simulink model "BoostQSim2018a"  (R2018a)
settings: Solver=VariableStepAuto  StartTime=0.0  StopTime=Tsim  RelTol=1e-3
values from neighbouring files (symbols this model uses):
  BoostQ =     [Boost_Data.mat]
  BoostQParam =     [BoostQParameters.mat]
  DutyConst = BoostQParam.Dn    [BoostQ.m]
  Gains =     [Gains.mat]
  PRBS_Amp = .05    (= 0.05)    [BoostQ.m]    (also in BoostQPlms.m = 0.1; BoostQuadrat.m; QBoostPLMS.m)
  PRBS_N = 10    [BoostQ.m]    (also in BoostQPlms.m; BoostQuadrat.m; QBoostPLMS.m)
  PRBS_Ts = Tb    (= 0.002)    [BoostQ.m]    (also in BoostQPlms.m; BoostQuadrat.m; QBoostPLMS.m)
  Ramp_Max = 0.75    [BoostQ.m]    (also in BoostQPlms.m; BoostQuadrat.m; QBoostPLMS.m)
  Tsim = 1*Tsim_min    (= 2.046)    [BoostQ.m]    (also in BoostQPlms.m; BoostQuadrat.m; QBoostPLMS.m)
undefined symbols (not defined in the file or in its folder): RST_LPV, Unit
libraries: fl_lib x11, nesl_utility x8, pe_lib x5, powerlib_meascontrol x1
settings Model: Creator=marcus  LastModifiedBy=projeto

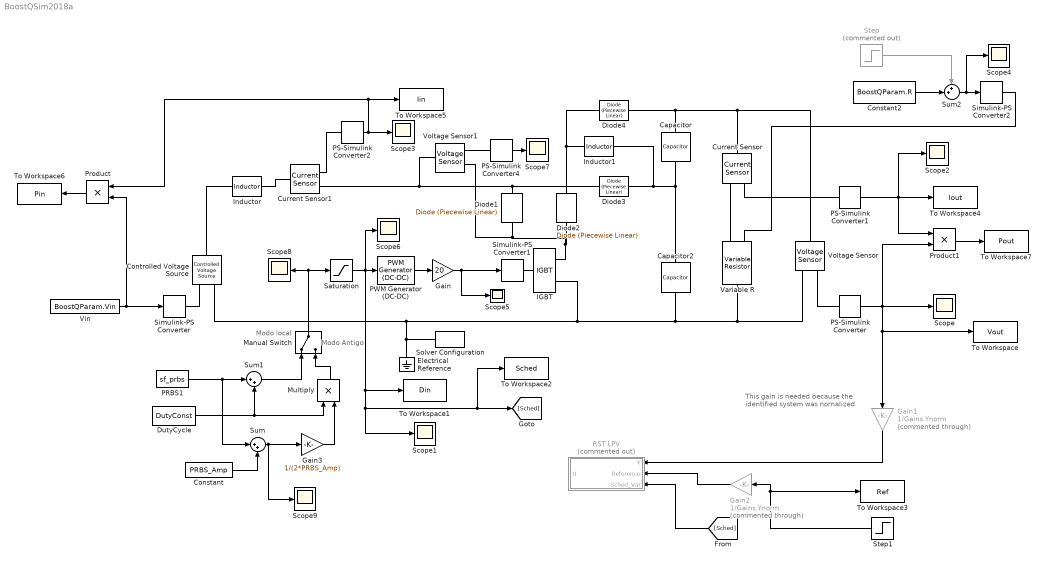
== system BoostQSim2018a ==
  note: Modo Antigo
  note: Modo local
  note: This gain is needed because
      | the identified system was nornalized
  Capacitor : fl_lib/Electrical/Electrical Elements/Capacitor  c=BoostQParam.C1 F  r=BoostQParam.rC1 Ohm  g=0 1/Ohm  i_specify=off  i_priority=None  i=0 A  i_nominal_specify=off  i_nominal_unit=A  i_nominal_value=1  v_specify=off  v_priority=None  v=0 V  v_nominal_specify=off  v_nominal_unit=V  v_nominal_value=1  vc_specify=off  vc_priority=High  vc=0 V  vc_nominal_specify=off  vc_nominal_unit=V  vc_nominal_value=1
  Capacitor2 : fl_lib/Electrical/Electrical Elements/Capacitor  c=BoostQParam.C2 F  r=BoostQParam.rC2 Ohm  g=0 1/Ohm  i_specify=off  i_priority=None  i=0 A  i_nominal_specify=off  i_nominal_unit=A  i_nominal_value=1  v_specify=off  v_priority=None  v=0 V  v_nominal_specify=off  v_nominal_unit=V  v_nominal_value=1  vc_specify=on  vc_priority=High  vc=BoostQParam.Vin V  vc_nominal_specify=off  vc_nominal_unit=V  vc_nominal_value=1
  Constant : Constant  Value=PRBS_Amp
  Constant2 : Constant  Value=BoostQParam.R
  Controlled Voltage Source : fl_lib/Electrical/Electrical Sources/Controlled Voltage Source
  Current Sensor : fl_lib/Electrical/Electrical Sensors/Current Sensor
  Current Sensor1 : fl_lib/Electrical/Electrical Sensors/Current Sensor
  Diode{1..4} (4 alike) : pe_lib/Semiconductors/Fundamental Components/Diode (Piecewise Linear)  Vf=0.01 V  Ron=0.01 Ohm  Goff=1e-5 1/Ohm  N_series=1  N_parallel=1
      settings: SourceProductName=Simscape Electrical  SourceProductBaseCode=PS
  DutyCycle : Constant  Value=DutyConst
  Electrical Reference : fl_lib/Electrical/Electrical Elements/Electrical Reference
  Gain : Gain  Gain=20
  Gain1 : Gain  Commented=through  Gain=1/Gains.Ynorm
  Gain2 : Gain  Commented=through  Gain=1/Gains.Ynorm
  Gain3 : Gain  Gain=1/(2*PRBS_Amp)
  IGBT : pe_lib/Semiconductors/Fundamental Components/IGBT  Vf=0.8 V  Ron=0.001 Ohm  Goff=1e-5 1/Ohm  Vth=6 V  diode_param=1  diode_Vf=0.8 V  diode_Ron=0.001 Ohm  diode_Goff=1e-5 1/Ohm  diode_C=5e-8 F  diode_iRM=-235 A  diode_iF=300 A  diode_idot=-50 A/us  diode_trr_param=1  diode_trr_factor=3  diode_trr=15 us  diode_Qrr=1.5e+3 s*uA  thermal_loss_option=2  Voff=300 V  Tau=1e-4 s  Tj=[ 298.15 398.15 ] K  Iout_scalar=600 A  Eon_scalar=0.02286 J  Eoff_scalar=0.01714 J  Von_scalar=2.7 V  Iout_data=[ 0 10 50 100 200 400 600 ] A  Eon_data=[ 0 2.9e-4 0.00143 0.00286 0.00571 0.01314 0.02286; 0 5.7e-4 0.00263 0.00514 0.01029 0.02057 0.03029 ] J  Eoff_data=[ 0 2.1e-4 0.00107 0.00214 0.00429 0.009859999999999999 0.01714; 0 4.3e-4 0.00197 0.00386 0.00771 0.01543 0.02271 ] J  Von_data=[ 0 1.1 1.3 1.45 1.75 2.25 2.7; 0 1 1.15 1.35 1.7 2.35 3 ] V
      settings: SourceProductName=Simscape Electrical  SourceProductBaseCode=PS
  Inductor : fl_lib/Electrical/Electrical Elements/Inductor  l=BoostQParam.L1 H  r=BoostQParam.rL1 Ohm  g=1e-9 1/Ohm  i_specify=off  i_priority=None  i=0 A  i_nominal_specify=off  i_nominal_unit=A  i_nominal_value=1  v_specify=off  v_priority=None  v=0 V  v_nominal_specify=off  v_nominal_unit=V  v_nominal_value=1  i_L_specify=off  i_L_priority=High  i_L=0 A  i_L_nominal_specify=off  i_L_nominal_unit=A  i_L_nominal_value=1
  Inductor1 : fl_lib/Electrical/Electrical Elements/Inductor  l=BoostQParam.L2 H  r=BoostQParam.rL2 Ohm  g=1e-9 1/Ohm  i_specify=off  i_priority=None  i=0 A  i_nominal_specify=off  i_nominal_unit=A  i_nominal_value=1  v_specify=off  v_priority=None  v=0 V  v_nominal_specify=off  v_nominal_unit=V  v_nominal_value=1  i_L_specify=off  i_L_priority=High  i_L=0 A  i_L_nominal_specify=off  i_L_nominal_unit=A  i_L_nominal_value=1
  Manual Switch : ManualSwitch
  Multiply : Product
  PRBS1 : S-Function  FunctionName=sf_prbs  Parameters=K,N,Ts  SFunctionDeploymentMode=off  EnableBusSupport=off  mask{K=PRBS_Amp, N=PRBS_N, Ts=PRBS_Ts}
      mask prompts: K "Ganho (K):"; N "Número de Células (usar 5, 7 ou 10):"; Ts "Tempo de amostragem (seg):"
      mask Display: disp('P R B S')
  PS-Simulink Converter{,1..2,4} (4 alike) : nesl_utility/PS-Simulink Converter  PhysicalDomain=network_engine_domain  SubClassName=ps_output  LeftPortType=input  RightPortType=output  PseudoPeriodic=off  Frequencies=[]  Unit=1  AffineConversion=off
  PWM Generator (DC-DC) : powerlib_meascontrol/Pulse & Signal Generators/PWM Generator (DC-DC)  Fsw=BoostQParam.f  Ts=0
      settings: SourceProductName=Simscape Electrical
  Product : Product
  Product1 : Product
  RST LPV : Subsystem  Commented=on
  Saturation : Saturate  UpperLimit=Ramp_Max*1.2  LowerLimit=0
  Scope{,1..9} (10 alike) : Scope
  Simulink-PS Converter : nesl_utility/Simulink-PS Converter  PhysicalDomain=network_engine_domain  SubClassName=ps_input  LeftPortType=input  RightPortType=output  PseudoPeriodic=off  Frequencies=[]  NoiseDistribution=none  NoiseParameters=[]  Unit=1  AffineConversion=off  FilteringAndDerivatives=provide  SimscapeFilterOrder=1  InputFilterTimeConstant=0.001  UdotUserProvided=0
  Simulink-PS Converter1 : nesl_utility/Simulink-PS Converter  PhysicalDomain=network_engine_domain  SubClassName=ps_input  LeftPortType=input  RightPortType=output  PseudoPeriodic=off  Frequencies=[]  NoiseDistribution=none  NoiseParameters=[]  Unit=1  AffineConversion=off  FilteringAndDerivatives=provide  SimscapeFilterOrder=1  InputFilterTimeConstant=0.001  UdotUserProvided=0
  Simulink-PS Converter2 : nesl_utility/Simulink-PS Converter  PhysicalDomain=network_engine_domain  SubClassName=ps_input  LeftPortType=input  RightPortType=output  PseudoPeriodic=off  Frequencies=[]  NoiseDistribution=none  NoiseParameters=[]  Unit=1  AffineConversion=off  FilteringAndDerivatives=zero  SimscapeFilterOrder=1  InputFilterTimeConstant=0.001  UdotUserProvided=0
  Solver Configuration : nesl_utility/Solver Configuration  PhysicalDomain=network_engine_domain  SubClassName=solver  LeftPortType=input  RightPortType=generic  Tones=[]  Harmonics=[]  SimulateNoise=off  Profile=off  UseLocalSampling=off  EnableSwitchedLinearOptims=on  FrequencyDomain=off  UseCCode=off  RelTol=0.001  AbsTol=1e-06  MinStep=1e-09  ToWorkspace=off  RevertToSquareIcSolve=off  NumHomotopyIterations=100  PhasorMode=off  PhasorModeNumHarmonics=1  DoDC=off  ResidualTolerance=1e-09  UseLocalSolver=off  LocalSolverChoice=NE_BACKWARD_EULER_ADVANCER  LocalSolverSampleTime=0.001  DoFixedCost=off  MaxNonlinIter=3  MaxModeIter=2  LinearAlgebra=Sparse  EquationFormulation=NE_TIME_EF  DelaysMemoryBudget=1024  AutomaticFiltering=on  FilteringTimeConstant=0.001  PartitionStorageMethod=AS_NEEDED  PartitionMemoryBudget=1024
  Step : Step  Commented=on  SampleTime=0
  Step1 : Step  Time=Tsim/3  Before=50  After=80  SampleTime=0
  Sum : Sum  Inputs=|++
  Sum1 : Sum  Inputs=|++
  Sum2 : Sum  Inputs=++|
  To Workspace : ToWorkspace  VariableName=Vout  SaveFormat=Timeseries  SampleTime=BoostQParam.Ts
  To Workspace1 : ToWorkspace  VariableName=Din  SaveFormat=Timeseries  SampleTime=BoostQParam.Ts
  To Workspace2 : ToWorkspace  VariableName=Sched  SaveFormat=Timeseries  SampleTime=BoostQParam.Ts
  To Workspace3 : ToWorkspace  VariableName=Ref  SaveFormat=Timeseries  SampleTime=BoostQParam.Ts
  To Workspace4 : ToWorkspace  VariableName=Iout  SaveFormat=Timeseries  SampleTime=BoostQParam.Ts
  To Workspace5 : ToWorkspace  VariableName=Iin  SaveFormat=Timeseries  SampleTime=BoostQParam.Ts
  To Workspace6 : ToWorkspace  VariableName=Pin  SaveFormat=Timeseries  SampleTime=BoostQParam.Ts
  To Workspace7 : ToWorkspace  VariableName=Pout  SaveFormat=Timeseries  SampleTime=BoostQParam.Ts
  Variable R : fl_lib/Electrical/Electrical Elements/Variable Resistor  Rmin=0 Ohm  i_specify=off  i_priority=None  i=0 A  i_nominal_specify=off  i_nominal_unit=A  i_nominal_value=1  v_specify=off  v_priority=None  v=0 V  v_nominal_specify=off  v_nominal_unit=V  v_nominal_value=1
  Vin : Constant  Value=BoostQParam.Vin
  Voltage Sensor : fl_lib/Electrical/Electrical Sensors/Voltage Sensor
  Voltage Sensor1 : fl_lib/Electrical/Electrical Sensors/Voltage Sensor
  wires:
  Vin/1 -> Product/2, Simulink-PS Converter/1
  PWM Generator (DC-DC)/1 -> Gain/1
  Constant2/1 -> Sum2/2
  Step/1 -> Sum2/1
  PS-Simulink Converter1/1 -> Product1/1, Scope2/1, To Workspace4/1
  PS-Simulink Converter2/1 -> Scope3/1, To Workspace5/1, Product/1
  [Sched] -> RST LPV/3(Sched_Var)
  Gain1/1 -> RST LPV/1(Y)
  Step1/1 -> Gain2/1, To Workspace3/1
  Gain2/1 -> RST LPV/2(Reference)
  Sum2/1 -> Scope4/1, Simulink-PS Converter2/1
  Product/1 -> To Workspace6/1
  Product1/1 -> To Workspace7/1
  PS-Simulink Converter4/1 -> Scope7/1
  Gain/1 -> Simulink-PS Converter1/1, Scope5/1
  PS-Simulink Converter/1 -> Scope/1, Product1/2, To Workspace/1, Gain1/1
  Manual Switch/1 -> Saturation/1, Scope8/1
  Saturation/1 -> Scope6/1, PWM Generator (DC-DC)/1, Scope1/1, To Workspace2/1, [Sched], To Workspace1/1
  PRBS1/1 -> Sum/1, Sum1/1
  DutyCycle/1 -> Sum1/2, Multiply/1
  Sum1/1 -> Manual Switch/1
  Constant/1 -> Sum/2
  Sum/1 -> Scope9/1, Gain3/1
  Gain3/1 -> Multiply/2
  Multiply/1 -> Manual Switch/2
  connections:
  Inductor/LConn1 -- Controlled Voltage Source/LConn1
  Simulink-PS Converter/RConn1 -- Controlled Voltage Source/RConn1
  Controlled Voltage Source/RConn2 -- Capacitor2/RConn1 -- Voltage Sensor/RConn2 -- Variable R/RConn1 -- IGBT/RConn2 -- Solver Configuration/RConn1 -- Electrical Reference/LConn1
  IGBT/LConn1 -- Simulink-PS Converter1/RConn1
  Current Sensor1/RConn2 -- Voltage Sensor1/LConn1 -- Diode1/LConn1 -- Diode3/LConn1
  Diode1/RConn1 -- Voltage Sensor1/RConn2 -- Diode2/RConn1 -- IGBT/RConn1
  Simulink-PS Converter2/RConn1 -- Variable R/LConn1
  Diode3/RConn1 -- Inductor1/RConn1 -- Capacitor/RConn1 -- Capacitor2/LConn1
  Diode4/RConn1 -- Current Sensor/LConn1 -- Voltage Sensor/LConn1 -- Capacitor/LConn1
  Diode4/LConn1 -- Diode2/LConn1 -- Inductor1/LConn1
  Voltage Sensor/RConn1 -- PS-Simulink Converter/LConn1
  Current Sensor/RConn2 -- Variable R/LConn2
  PS-Simulink Converter1/LConn1 -- Current Sensor/RConn1
  Current Sensor1/LConn1 -- Inductor/RConn1
  PS-Simulink Converter2/LConn1 -- Current Sensor1/RConn1
  PS-Simulink Converter4/LConn1 -- Voltage Sensor1/RConn1

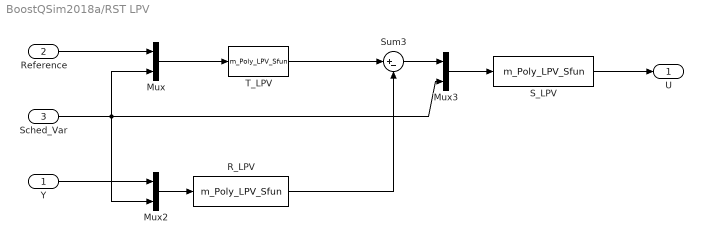
== system BoostQSim2018a/RST LPV ==
  Y : Inport
  Reference : Inport  Port=2
  Sched_Var : Inport  Port=3
  Mux : Mux  Inputs=2
  Mux2 : Mux  Inputs=2
  Mux3 : Mux  Inputs=2
  R_LPV : S-Function  FunctionName=m_Poly_LPV_Sfun  Parameters=BoostQ.Ts,Unit,RST_LPV.R  SFunctionDeploymentMode=off  EnableBusSupport=off
  S_LPV : S-Function  FunctionName=m_Poly_LPV_Sfun  Parameters=BoostQ.Ts,RST_LPV.S,Unit  SFunctionDeploymentMode=off  EnableBusSupport=off
  Sum3 : Sum  Inputs=|+-
  T_LPV : S-Function  FunctionName=m_Poly_LPV_Sfun  Parameters=BoostQ.Ts,Unit,RST_LPV.T  SFunctionDeploymentMode=off  EnableBusSupport=off
  U : Outport
  wires:
  Mux/1 -> T_LPV/1
  Reference/1 -> Mux/1
  Sched_Var/1 -> Mux2/2, Mux3/2, Mux/2
  Y/1 -> Mux2/1
  Mux2/1 -> R_LPV/1
  R_LPV/1 -> Sum3/2
  Sum3/1 -> Mux3/1
  Mux3/1 -> S_LPV/1
  S_LPV/1 -> U/1
  T_LPV/1 -> Sum3/1
